simulink model "FrequencyModel"  (R2023a)
settings: Solver=VariableStepAuto  StartTime=0.0  StopTime=Tt+T-Ts  RelTol=1e-3
values from neighbouring files (symbols this model uses):
  N = 200    [Init.m]    (also in frequencyData.mat)
  Ts = 0.01    [Init.m]    (also in frequencyData.mat)
  wr = 2*pi/T    (= 0.628318530718)    [Init.m]    (also in frequencyData.mat)
settings Model: Creator=quarc_user  LastModifiedBy=quarc_user

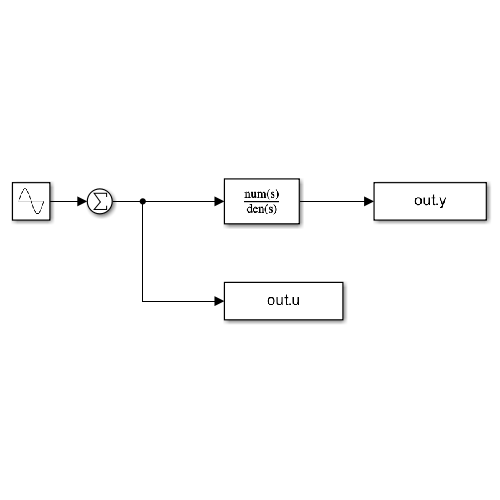
[thumbnail: Simulink's stored preview of the top-level diagram]
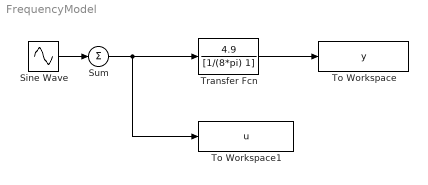
== system FrequencyModel ==
  Sine Wave : Sin  Amplitude=2  Frequency=[1:N]*wr  Phase=2*pi*rand(1,N)  SampleTime=0
  Sum : Sum  Inputs=+
  To Workspace : ToWorkspace  VariableName=y  SaveFormat=Timeseries  SampleTime=Ts
      settings: MaxDataPoints=T/Ts
  To Workspace1 : ToWorkspace  VariableName=u  SaveFormat=Timeseries  SampleTime=Ts
      settings: MaxDataPoints=T/Ts
  Transfer Fcn : TransferFcn  Numerator=[4.9]  Denominator=[1/(8*pi) 1]
  wires:
  Sine Wave/1 -> Sum/1
  Transfer Fcn/1 -> To Workspace/1
  Sum/1 -> To Workspace1/1, Transfer Fcn/1
